simulink model "control_pos_3dof_sinMI"  (R2023b)
settings: Solver=ode5  StartTime=0.0  StopTime=tsim  FixedStep=tstep  RelTol=1e-3
undefined symbols (not defined in the file): a0, a1, robot_params, t_qeq_init, t_tr_init, tau_L
(part 1 of 2)
settings Model: Creator=HP  LastModifiedBy=HP

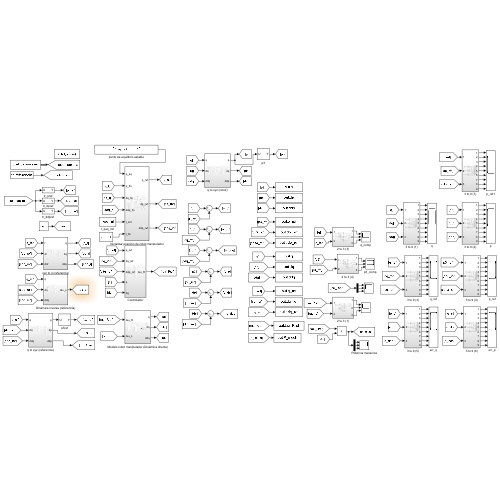
[thumbnail: Simulink's stored preview of the top-level diagram]
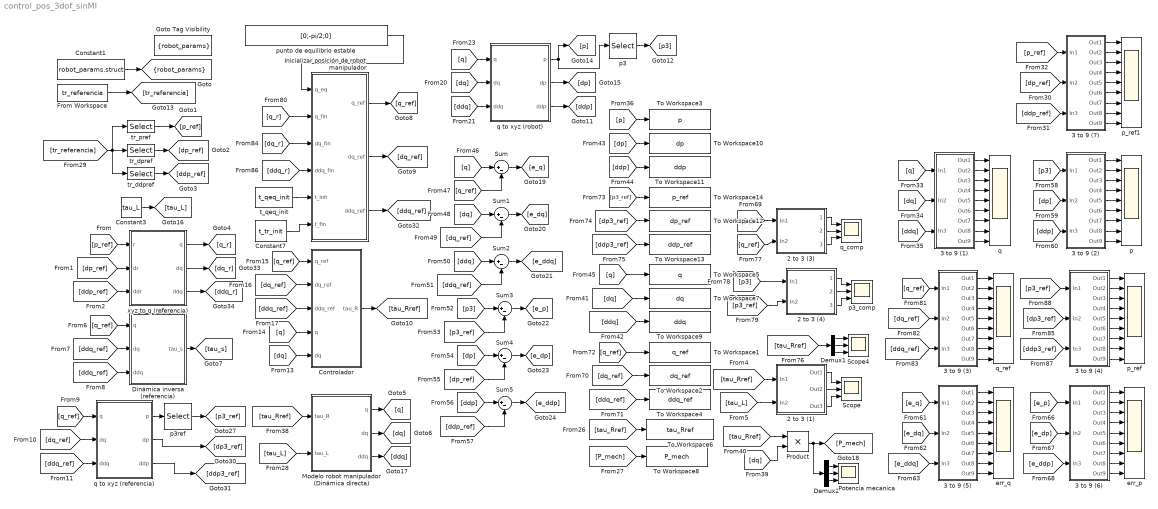
== system control_pos_3dof_sinMI ==
  2 to 3 (1) : Subsystem
  2 to 3 (3) : Subsystem
  2 to 3 (4) : Subsystem
  3 to 9 (1) : Subsystem
  3 to 9 (2) : Subsystem
  3 to 9 (3) : Subsystem
  3 to 9 (4) : Subsystem
  3 to 9 (5) : Subsystem
  3 to 9 (6) : Subsystem
  3 to 9 (7) : Subsystem
  Constant1 : Constant  Value=robot_params.struct  OutDataTypeStr=Bus: robot_params_bus
  Constant3 : Constant  Value=tau_L
  Constant7 : Constant  Value=t_tr_init
  Controlador : Subsystem
  Demux1 : Demux  Outputs=3
  Demux2 : Demux  Outputs=3
  Dinámica inversa (referencia) : Subsystem
  From Workspace : FromWorkspace  VariableName=tr_referencia
  Goto Tag Visibility : GotoTagVisibility  GotoTag=robot_params
  Inicializar posición de robot manipulador : Subsystem
  Modelo robot manipulador (Dinámica directa) : Subsystem
  Potencia mecanica : Scope  NumInputPorts=3
  Product : Product
  Scope : Scope  NumInputPorts=3
  Scope4 : Scope  NumInputPorts=3
  Sum{,1..5} (6 alike) : Sum  Inputs=|+-
  To Workspace1 : ToWorkspace  VariableName=q_ref  SaveFormat=Timeseries  SampleTime=-1
  To Workspace10 : ToWorkspace  VariableName=dp  SaveFormat=Timeseries  SampleTime=-1
  To Workspace11 : ToWorkspace  VariableName=ddp  SaveFormat=Timeseries  SampleTime=-1
  To Workspace12 : ToWorkspace  VariableName=dp_ref  SaveFormat=Timeseries  SampleTime=-1
  To Workspace13 : ToWorkspace  VariableName=ddp_ref  SaveFormat=Timeseries  SampleTime=-1
  To Workspace14 : ToWorkspace  VariableName=p_ref  SaveFormat=Timeseries  SampleTime=-1
  To Workspace2 : ToWorkspace  VariableName=dq_ref  SaveFormat=Timeseries  SampleTime=-1
  To Workspace3 : ToWorkspace  VariableName=p  SaveFormat=Timeseries  SampleTime=-1
  To Workspace4 : ToWorkspace  VariableName=ddq_ref  SaveFormat=Timeseries  SampleTime=-1
  To Workspace5 : ToWorkspace  VariableName=q  SaveFormat=Timeseries  SampleTime=-1
  To Workspace6 : ToWorkspace  VariableName=tau_Rref  SaveFormat=Timeseries  SampleTime=-1
  To Workspace7 : ToWorkspace  VariableName=dq  SaveFormat=Timeseries  SampleTime=-1
  To Workspace8 : ToWorkspace  VariableName=P_mech  SaveFormat=Timeseries  SampleTime=-1
  To Workspace9 : ToWorkspace  VariableName=ddq  SaveFormat=Timeseries  SampleTime=-1
  err_p : Scope  NumInputPorts=9
  err_q : Scope  NumInputPorts=9
  p : Scope  NumInputPorts=9
  p3 : Selector  NumberOfDimensions=2  InputPortWidth=3  IndexOptions=Index vector (dialog),Index vector (dialog)  Indices=[1:3],3  OutputSizes=1,1
  p3_comp : Scope  NumInputPorts=3
  p3ref : Selector  NumberOfDimensions=2  InputPortWidth=3  IndexOptions=Index vector (dialog),Index vector (dialog)  Indices=[1:3],3  OutputSizes=1,1
  p_ref : Scope  NumInputPorts=9
  p_ref1 : Scope  NumInputPorts=9
  punto de equilibrio estable : Constant  Value=[0;-pi/2;0]
  q : Scope  NumInputPorts=9
  q to xyz (referencia) : Subsystem
  q to xyz (robot) : Subsystem
  q_comp : Scope  NumInputPorts=3
  q_ref : Scope  NumInputPorts=9
  t_qeq_init : Constant  Value=t_qeq_init
  tr_ddpref : Selector  NumberOfDimensions=2  InputPortWidth=3  IndexOptions=Index vector (dialog),Index vector (dialog)  Indices=[7:9],1  OutputSizes=1,1
  tr_dpref : Selector  NumberOfDimensions=2  InputPortWidth=3  IndexOptions=Index vector (dialog),Index vector (dialog)  Indices=[4:6],1  OutputSizes=1,1
  tr_pref : Selector  NumberOfDimensions=2  InputPortWidth=3  IndexOptions=Index vector (dialog),Index vector (dialog)  Indices=[1:3],1  OutputSizes=1,1
  xyz to q (referencia) : Subsystem
  tag scope: robot_params=scoped
  wires:
  From Workspace/1 -> [tr_referencia]
  Constant1/1 -> [robot_params]
  Constant3/1 -> [tau_L]
  [q_ref] -> Dinámica inversa (referencia)/1(q)
  [ddq_ref] -> Dinámica inversa (referencia)/2(dq)
  [ddq_ref] -> Dinámica inversa (referencia)/3(ddq)
  Dinámica inversa (referencia)/1(tau_s) -> [tau_s]
  [q_ref] -> Controlador/1(q_ref)
  [dq_ref] -> Controlador/2(dq_ref)
  [ddq_ref] -> Controlador/3(ddq_ref)
  [q] -> Controlador/4(q)
  [dq] -> Controlador/5(dq)
  Controlador/1(tau_R) -> [tau_Rref]
  [tr_referencia] -> tr_ddpref/1, tr_pref/1, tr_dpref/1
  tr_pref/1 -> [p_ref]
  tr_dpref/1 -> [dp_ref]
  tr_ddpref/1 -> [ddp_ref]
  3 to 9 (5)/3(Out3) -> err_q/3
  3 to 9 (2)/5(Out5) -> p/5
  3 to 9 (3)/9(Out9) -> q_ref/9
  3 to 9 (6)/5(Out5) -> err_p/5
  3 to 9 (5)/4(Out4) -> err_q/4
  3 to 9 (7)/8(Out8) -> p_ref1/8
  3 to 9 (4)/3(Out3) -> p_ref/3
  3 to 9 (1)/1(Out1) -> q/1
  [dp3_ref] -> 3 to 9 (4)/2(In2)
  3 to 9 (3)/2(Out2) -> q_ref/2
  [dq] -> To Workspace7/1
  2 to 3 (4)/2(2) -> p3_comp/2
  [ddq_ref] -> 3 to 9 (3)/3(In3)
  [dp] -> Sum4/1
  3 to 9 (1)/9(Out9) -> q/9
  [ddp] -> 3 to 9 (2)/3(In3)
  3 to 9 (2)/8(Out8) -> p/8
  3 to 9 (2)/1(Out1) -> p/1
  [dp] -> 3 to 9 (2)/2(In2)
  [q_ref] -> 2 to 3 (3)/2(In2)
  2 to 3 (3)/2(2) -> q_comp/2
  3 to 9 (4)/5(Out5) -> p_ref/5
  [q] -> 2 to 3 (3)/1(In1)
  [ddp_ref] -> 3 to 9 (7)/3(In3)
  [ddq] -> 3 to 9 (1)/3(In3)
  3 to 9 (2)/3(Out3) -> p/3
  3 to 9 (1)/2(Out2) -> q/2
  3 to 9 (2)/4(Out4) -> p/4
  3 to 9 (4)/6(Out6) -> p_ref/6
  3 to 9 (6)/1(Out1) -> err_p/1
  [p3_ref] -> 3 to 9 (4)/1(In1)
  3 to 9 (1)/3(Out3) -> q/3
  [ddp3_ref] -> 3 to 9 (4)/3(In3)
  3 to 9 (1)/8(Out8) -> q/8
  3 to 9 (7)/9(Out9) -> p_ref1/9
  3 to 9 (7)/1(Out1) -> p_ref1/1
  3 to 9 (4)/4(Out4) -> p_ref/4
  3 to 9 (5)/1(Out1) -> err_q/1
  3 to 9 (2)/2(Out2) -> p/2
  3 to 9 (6)/4(Out4) -> err_p/4
  [ddp] -> Sum5/1
  3 to 9 (7)/3(Out3) -> p_ref1/3
  [q] -> q to xyz (robot)/1(q)
  3 to 9 (3)/4(Out4) -> q_ref/4
  3 to 9 (7)/5(Out5) -> p_ref1/5
  2 to 3 (3)/1(1) -> q_comp/1
  3 to 9 (4)/7(Out7) -> p_ref/7
  [e_ddq] -> 3 to 9 (5)/3(In3)
  3 to 9 (1)/4(Out4) -> q/4
  3 to 9 (3)/3(Out3) -> q_ref/3
  [q_ref] -> To Workspace1/1
  3 to 9 (3)/5(Out5) -> q_ref/5
  [P_mech] -> To Workspace8/1
  3 to 9 (5)/6(Out6) -> err_q/6
  2 to 3 (4)/1(1) -> p3_comp/1
  3 to 9 (6)/7(Out7) -> err_p/7
  [e_q] -> 3 to 9 (5)/1(In1)
  3 to 9 (4)/1(Out1) -> p_ref/1
  3 to 9 (5)/8(Out8) -> err_q/8
  [tau_Rref] -> Demux1/1
  3 to 9 (2)/7(Out7) -> p/7
  Sum5/1 -> [e_ddp]
  Demux2/3 -> Potencia mecanica/3
  3 to 9 (4)/8(Out8) -> p_ref/8
  3 to 9 (6)/2(Out2) -> err_p/2
  [tau_Rref] -> To Workspace6/1
  [e_dp] -> 3 to 9 (6)/2(In2)
  [p3] -> 2 to 3 (4)/1(In1)
  3 to 9 (5)/7(Out7) -> err_q/7
  3 to 9 (3)/1(Out1) -> q_ref/1
  [ddq] -> Sum2/1
  3 to 9 (2)/9(Out9) -> p/9
  3 to 9 (3)/6(Out6) -> q_ref/6
  3 to 9 (4)/9(Out9) -> p_ref/9
  3 to 9 (3)/8(Out8) -> q_ref/8
  3 to 9 (1)/7(Out7) -> q/7
  [ddq_ref] -> Sum2/2
  [dp3_ref] -> To Workspace12/1
  2 to 3 (1)/3(Out3) -> Scope/3
  2 to 3 (4)/3(3) -> p3_comp/3
  3 to 9 (4)/2(Out2) -> p_ref/2
  [dq_ref] -> 3 to 9 (3)/2(In2)
  3 to 9 (6)/3(Out3) -> err_p/3
  [dq] -> Product/2
  3 to 9 (5)/5(Out5) -> err_q/5
  [e_p] -> 3 to 9 (6)/1(In1)
  [dq] -> 3 to 9 (1)/2(In2)
  [dq] -> Sum1/1
  [p_ref] -> 3 to 9 (7)/1(In1)
  Sum/1 -> [e_q]
  3 to 9 (5)/9(Out9) -> err_q/9
  3 to 9 (7)/4(Out4) -> p_ref1/4
  3 to 9 (7)/6(Out6) -> p_ref1/6
  [dp_ref] -> 3 to 9 (7)/2(In2)
  Demux1/1 -> Scope4/1
  2 to 3 (3)/3(3) -> q_comp/3
  [q_ref] -> 3 to 9 (3)/1(In1)
  Sum2/1 -> [e_ddq]
  Demux1/2 -> Scope4/2
  [tau_L] -> 2 to 3 (1)/2(In2)
  Demux2/2 -> Potencia mecanica/2
  [p3] -> 3 to 9 (2)/1(In1)
  q to xyz (robot)/1(p) -> p3/1, [p]
  3 to 9 (6)/8(Out8) -> err_p/8
  [q_ref] -> Sum/2
  3 to 9 (6)/6(Out6) -> err_p/6
  3 to 9 (1)/6(Out6) -> q/6
  [dp] -> To Workspace10/1
  Demux1/3 -> Scope4/3
  3 to 9 (7)/7(Out7) -> p_ref1/7
  [p] -> To Workspace3/1
  [ddq_ref] -> To Workspace4/1
  Sum3/1 -> [e_p]
  Sum4/1 -> [e_dp]
  [p3] -> Sum3/1
  [dq_ref] -> Sum1/2
  3 to 9 (2)/6(Out6) -> p/6
  Sum1/1 -> [e_dq]
  [tau_Rref] -> 2 to 3 (1)/1(In1)
  Demux2/1 -> Potencia mecanica/1
  [e_dq] -> 3 to 9 (5)/2(In2)
  [q] -> Sum/1
  [dp_ref] -> Sum4/2
  3 to 9 (5)/2(Out2) -> err_q/2
  [ddq] -> q to xyz (robot)/3(ddq)
  [e_ddp] -> 3 to 9 (6)/3(In3)
  [ddp_ref] -> Sum5/2
  [p3_ref] -> Sum3/2
  3 to 9 (3)/7(Out7) -> q_ref/7
  [p3_ref] -> 2 to 3 (4)/2(In2)
  p3/1 -> [p3]
  2 to 3 (1)/1(Out1) -> Scope/1
  [dq] -> q to xyz (robot)/2(dq)
  [ddp3_ref] -> To Workspace13/1
  3 to 9 (1)/5(Out5) -> q/5
  [ddq] -> To Workspace9/1
  [p3_ref] -> To Workspace14/1
  [ddp] -> To Workspace11/1
  3 to 9 (6)/9(Out9) -> err_p/9
  q to xyz (robot)/3(ddp) -> [ddp]
  [q] -> 3 to 9 (1)/1(In1)
  [q] -> To Workspace5/1
  q to xyz (robot)/2(dp) -> [dp]
  [dq_ref] -> To Workspace2/1
  Product/1 -> Demux2/1, [P_mech]
  [tau_Rref] -> Product/1
  3 to 9 (7)/2(Out2) -> p_ref1/2
  2 to 3 (1)/2(Out2) -> Scope/2
  xyz to q (referencia)/1(q) -> [q_r]
  xyz to q (referencia)/2(dq) -> [dq_r]
  [ddp_ref] -> xyz to q (referencia)/3(ddr)
  [p_ref] -> xyz to q (referencia)/1(r)
  [dp_ref] -> xyz to q (referencia)/2(dr)
  xyz to q (referencia)/3(ddq) -> [ddq_r]
  [dq_ref] -> q to xyz (referencia)/2(dq)
  q to xyz (referencia)/2(dp) -> [dp3_ref]
  q to xyz (referencia)/3(ddp) -> [ddp3_ref]
  [ddq_ref] -> q to xyz (referencia)/3(ddq)
  Modelo robot manipulador (Dinámica directa)/3(ddq) -> [ddq]
  [tau_L] -> Modelo robot manipulador (Dinámica directa)/2(tau_L)
  Modelo robot manipulador (Dinámica directa)/1(q) -> [q]
  Modelo robot manipulador (Dinámica directa)/2(dq) -> [dq]
  [tau_Rref] -> Modelo robot manipulador (Dinámica directa)/1(tau_R)
  [q_ref] -> q to xyz (referencia)/1(q)
  q to xyz (referencia)/1(p) -> p3ref/1
  p3ref/1 -> [p3_ref]
  Constant7/1 -> Inicializar posición de robot manipulador/6(t_fin)
  [dq_r] -> Inicializar posición de robot manipulador/3(dq_fin)
  [q_r] -> Inicializar posición de robot manipulador/2(q_fin)
  [ddq_r] -> Inicializar posición de robot manipulador/4(ddq_fin)
  t_qeq_init/1 -> Inicializar posición de robot manipulador/5(t_init)
  Inicializar posición de robot manipulador/3(ddq_ref) -> [ddq_ref]
  punto de equilibrio estable/1 -> Inicializar posición de robot manipulador/1(q_eq)
  Inicializar posición de robot manipulador/1(q_ref) -> [q_ref]
  Inicializar posición de robot manipulador/2(dq_ref) -> [dq_ref]

== system control_pos_3dof_sinMI/2 to 3 (1) ==
  In1 : Inport
  In2 : Inport  Port=2
  Demux : Demux  Outputs=3
  Demux1 : Demux  Outputs=3
  Mux : Mux  Inputs=2
  Mux1 : Mux  Inputs=2
  Mux2 : Mux  Inputs=2
  Out1 : Outport
  Out2 : Outport  Port=2
  Out3 : Outport  Port=3
  wires:
  Demux/3 -> Mux2/1
  Mux2/1 -> Out3/1
  Mux1/1 -> Out2/1
  Demux/1 -> Mux/1
  Demux1/1 -> Mux/2
  In1/1 -> Demux/1
  Demux/2 -> Mux1/1
  Demux1/2 -> Mux1/2
  Mux/1 -> Out1/1
  Demux1/3 -> Mux2/2
  In2/1 -> Demux1/1

== system control_pos_3dof_sinMI/2 to 3 (3) ==
  In1 : Inport
  In2 : Inport  Port=2
  Demux3 : Demux  Outputs=3
  Demux4 : Demux  Outputs=3
  Mux10 : Mux  Inputs=2
  Mux8 : Mux  Inputs=2
  Mux9 : Mux  Inputs=2
  1 : Outport
  2 : Outport  Port=2
  3 : Outport  Port=3
  wires:
  Demux4/3 -> Mux10/2
  Demux3/1 -> Mux8/1
  Demux3/2 -> Mux9/1
  Mux9/1 -> 2/1
  Demux4/2 -> Mux9/2
  Demux4/1 -> Mux8/2
  Demux3/3 -> Mux10/1
  Mux8/1 -> 1/1
  Mux10/1 -> 3/1
  In1/1 -> Demux3/1
  In2/1 -> Demux4/1

== system control_pos_3dof_sinMI/2 to 3 (4) ==
  In1 : Inport
  In2 : Inport  Port=2
  Demux3 : Demux  Outputs=3
  Demux4 : Demux  Outputs=3
  Mux10 : Mux  Inputs=2
  Mux8 : Mux  Inputs=2
  Mux9 : Mux  Inputs=2
  1 : Outport
  2 : Outport  Port=2
  3 : Outport  Port=3
  wires:
  Demux4/3 -> Mux10/2
  Demux3/1 -> Mux8/1
  Demux3/2 -> Mux9/1
  Mux9/1 -> 2/1
  Demux4/2 -> Mux9/2
  Demux4/1 -> Mux8/2
  Demux3/3 -> Mux10/1
  Mux8/1 -> 1/1
  Mux10/1 -> 3/1
  In1/1 -> Demux3/1
  In2/1 -> Demux4/1

== system control_pos_3dof_sinMI/3 to 9 (1) ==
  In1 : Inport
  In2 : Inport  Port=2
  In3 : Inport  Port=3
  Demux2 : Demux  Outputs=3
  Demux3 : Demux  Outputs=3
  Demux4 : Demux  Outputs=3
  Out1 : Outport
  Out2 : Outport  Port=2
  Out3 : Outport  Port=3
  Out4 : Outport  Port=4
  Out5 : Outport  Port=5
  Out6 : Outport  Port=6
  Out7 : Outport  Port=7
  Out8 : Outport  Port=8
  Out9 : Outport  Port=9
  wires:
  In3/1 -> Demux4/1
  Demux4/1 -> Out3/1
  Demux2/1 -> Out1/1
  Demux3/3 -> Out8/1
  Demux3/2 -> Out5/1
  Demux3/1 -> Out2/1
  In1/1 -> Demux2/1
  Demux2/3 -> Out7/1
  Demux4/3 -> Out9/1
  Demux4/2 -> Out6/1
  Demux2/2 -> Out4/1
  In2/1 -> Demux3/1

== system control_pos_3dof_sinMI/3 to 9 (2) ==
  In1 : Inport
  In2 : Inport  Port=2
  In3 : Inport  Port=3
  Demux2 : Demux  Outputs=3
  Demux3 : Demux  Outputs=3
  Demux4 : Demux  Outputs=3
  Out1 : Outport
  Out2 : Outport  Port=2
  Out3 : Outport  Port=3
  Out4 : Outport  Port=4
  Out5 : Outport  Port=5
  Out6 : Outport  Port=6
  Out7 : Outport  Port=7
  Out8 : Outport  Port=8
  Out9 : Outport  Port=9
  wires:
  In3/1 -> Demux4/1
  Demux4/1 -> Out3/1
  Demux2/1 -> Out1/1
  Demux3/3 -> Out8/1
  Demux3/2 -> Out5/1
  Demux3/1 -> Out2/1
  In1/1 -> Demux2/1
  Demux2/3 -> Out7/1
  Demux4/3 -> Out9/1
  Demux4/2 -> Out6/1
  Demux2/2 -> Out4/1
  In2/1 -> Demux3/1

== system control_pos_3dof_sinMI/3 to 9 (3) ==
  In1 : Inport
  In2 : Inport  Port=2
  In3 : Inport  Port=3
  Demux2 : Demux  Outputs=3
  Demux3 : Demux  Outputs=3
  Demux4 : Demux  Outputs=3
  Out1 : Outport
  Out2 : Outport  Port=2
  Out3 : Outport  Port=3
  Out4 : Outport  Port=4
  Out5 : Outport  Port=5
  Out6 : Outport  Port=6
  Out7 : Outport  Port=7
  Out8 : Outport  Port=8
  Out9 : Outport  Port=9
  wires:
  In3/1 -> Demux4/1
  Demux4/1 -> Out3/1
  Demux2/1 -> Out1/1
  Demux3/3 -> Out8/1
  Demux3/2 -> Out5/1
  Demux3/1 -> Out2/1
  In1/1 -> Demux2/1
  Demux2/3 -> Out7/1
  Demux4/3 -> Out9/1
  Demux4/2 -> Out6/1
  Demux2/2 -> Out4/1
  In2/1 -> Demux3/1

== system control_pos_3dof_sinMI/3 to 9 (4) ==
  In1 : Inport
  In2 : Inport  Port=2
  In3 : Inport  Port=3
  Demux2 : Demux  Outputs=3
  Demux3 : Demux  Outputs=3
  Demux4 : Demux  Outputs=3
  Out1 : Outport
  Out2 : Outport  Port=2
  Out3 : Outport  Port=3
  Out4 : Outport  Port=4
  Out5 : Outport  Port=5
  Out6 : Outport  Port=6
  Out7 : Outport  Port=7
  Out8 : Outport  Port=8
  Out9 : Outport  Port=9
  wires:
  In3/1 -> Demux4/1
  Demux4/1 -> Out3/1
  Demux2/1 -> Out1/1
  Demux3/3 -> Out8/1
  Demux3/2 -> Out5/1
  Demux3/1 -> Out2/1
  In1/1 -> Demux2/1
  Demux2/3 -> Out7/1
  Demux4/3 -> Out9/1
  Demux4/2 -> Out6/1
  Demux2/2 -> Out4/1
  In2/1 -> Demux3/1

== system control_pos_3dof_sinMI/3 to 9 (5) ==
  In1 : Inport
  In2 : Inport  Port=2
  In3 : Inport  Port=3
  Demux2 : Demux  Outputs=3
  Demux3 : Demux  Outputs=3
  Demux4 : Demux  Outputs=3
  Out1 : Outport
  Out2 : Outport  Port=2
  Out3 : Outport  Port=3
  Out4 : Outport  Port=4
  Out5 : Outport  Port=5
  Out6 : Outport  Port=6
  Out7 : Outport  Port=7
  Out8 : Outport  Port=8
  Out9 : Outport  Port=9
  wires:
  In3/1 -> Demux4/1
  Demux4/1 -> Out3/1
  Demux2/1 -> Out1/1
  Demux3/3 -> Out8/1
  Demux3/2 -> Out5/1
  Demux3/1 -> Out2/1
  In1/1 -> Demux2/1
  Demux2/3 -> Out7/1
  Demux4/3 -> Out9/1
  Demux4/2 -> Out6/1
  Demux2/2 -> Out4/1
  In2/1 -> Demux3/1

== system control_pos_3dof_sinMI/3 to 9 (6) ==
  In1 : Inport
  In2 : Inport  Port=2
  In3 : Inport  Port=3
  Demux2 : Demux  Outputs=3
  Demux3 : Demux  Outputs=3
  Demux4 : Demux  Outputs=3
  Out1 : Outport
  Out2 : Outport  Port=2
  Out3 : Outport  Port=3
  Out4 : Outport  Port=4
  Out5 : Outport  Port=5
  Out6 : Outport  Port=6
  Out7 : Outport  Port=7
  Out8 : Outport  Port=8
  Out9 : Outport  Port=9
  wires:
  In3/1 -> Demux4/1
  Demux4/1 -> Out3/1
  Demux2/1 -> Out1/1
  Demux3/3 -> Out8/1
  Demux3/2 -> Out5/1
  Demux3/1 -> Out2/1
  In1/1 -> Demux2/1
  Demux2/3 -> Out7/1
  Demux4/3 -> Out9/1
  Demux4/2 -> Out6/1
  Demux2/2 -> Out4/1
  In2/1 -> Demux3/1

== system control_pos_3dof_sinMI/3 to 9 (7) ==
  In1 : Inport
  In2 : Inport  Port=2
  In3 : Inport  Port=3
  Demux2 : Demux  Outputs=3
  Demux3 : Demux  Outputs=3
  Demux4 : Demux  Outputs=3
  Out1 : Outport
  Out2 : Outport  Port=2
  Out3 : Outport  Port=3
  Out4 : Outport  Port=4
  Out5 : Outport  Port=5
  Out6 : Outport  Port=6
  Out7 : Outport  Port=7
  Out8 : Outport  Port=8
  Out9 : Outport  Port=9
  wires:
  In3/1 -> Demux4/1
  Demux4/1 -> Out3/1
  Demux2/1 -> Out1/1
  Demux3/3 -> Out8/1
  Demux3/2 -> Out5/1
  Demux3/1 -> Out2/1
  In1/1 -> Demux2/1
  Demux2/3 -> Out7/1
  Demux4/3 -> Out9/1
  Demux4/2 -> Out6/1
  Demux2/2 -> Out4/1
  In2/1 -> Demux3/1

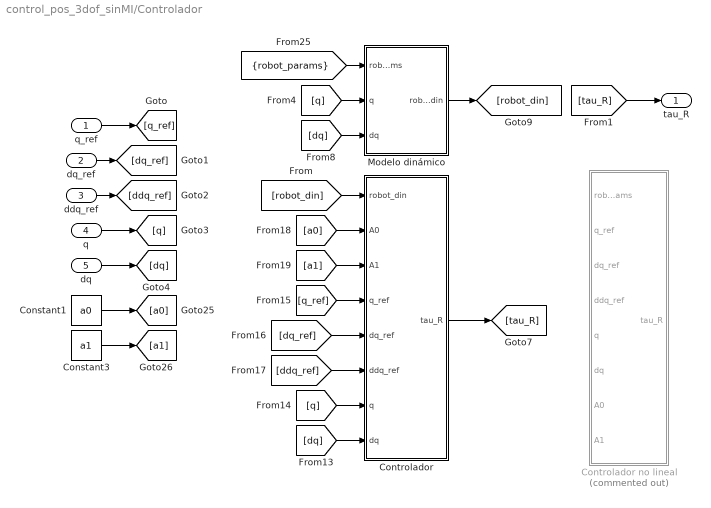
== system control_pos_3dof_sinMI/Controlador ==
  q_ref : Inport
  dq_ref : Inport  Port=2
  ddq_ref : Inport  Port=3
  q : Inport  Port=4
  dq : Inport  Port=5
  Constant1 : Constant  Value=a0
  Constant3 : Constant  Value=a1
  Controlador : MATLAB Function  TreatAsAtomicUnit=on
  Controlador no lineal : MATLAB Function  Commented=on  TreatAsAtomicUnit=on
  Modelo dinámico : MATLAB Function  TreatAsAtomicUnit=on
  tau_R : Outport
  wires:
  [dq] -> Modelo dinámico/3(dq)
  [q] -> Modelo dinámico/2(q)
  [robot_params] -> Modelo dinámico/1(robot_params)
  Modelo dinámico/1(robot_din) -> [robot_din]
  dq/1 -> [dq]
  q/1 -> [q]
  ddq_ref/1 -> [ddq_ref]
  dq_ref/1 -> [dq_ref]
  q_ref/1 -> [q_ref]
  [robot_din] -> Controlador/1(robot_din)
  [a0] -> Controlador/2(A0)
  [a1] -> Controlador/3(A1)
  [q_ref] -> Controlador/4(q_ref)
  [dq_ref] -> Controlador/5(dq_ref)
  [ddq_ref] -> Controlador/6(ddq_ref)
  [q] -> Controlador/7(q)
  [dq] -> Controlador/8(dq)
  Controlador/1(tau_R) -> [tau_R]
  [tau_R] -> tau_R/1
  Constant1/1 -> [a0]
  Constant3/1 -> [a1]

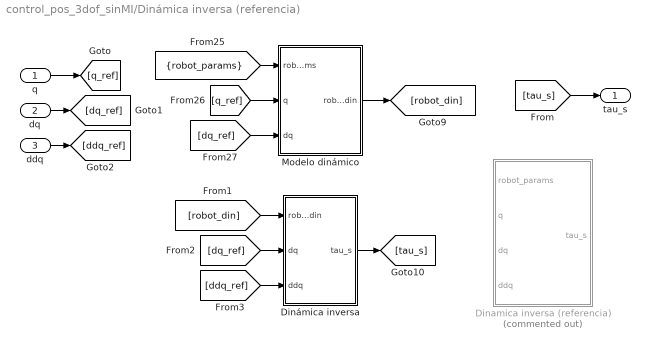
== system control_pos_3dof_sinMI/Dinámica inversa (referencia) ==
  q : Inport
  dq : Inport  Port=2
  ddq : Inport  Port=3
  Dinamica inversa (referencia) : MATLAB Function  Commented=on  TreatAsAtomicUnit=on
  Dinámica inversa : MATLAB Function  TreatAsAtomicUnit=on
  Modelo dinámico : MATLAB Function  TreatAsAtomicUnit=on
  tau_s : Outport
  wires:
  [dq_ref] -> Modelo dinámico/3(dq)
  [robot_params] -> Modelo dinámico/1(robot_params)
  Modelo dinámico/1(robot_din) -> [robot_din]
  [q_ref] -> Modelo dinámico/2(q)
  q/1 -> [q_ref]
  dq/1 -> [dq_ref]
  Dinámica inversa/1(tau_s) -> [tau_s]
  [robot_din] -> Dinámica inversa/1(robot_din)
  [ddq_ref] -> Dinámica inversa/3(ddq)
  [dq_ref] -> Dinámica inversa/2(dq)
  ddq/1 -> [ddq_ref]
  [tau_s] -> tau_s/1

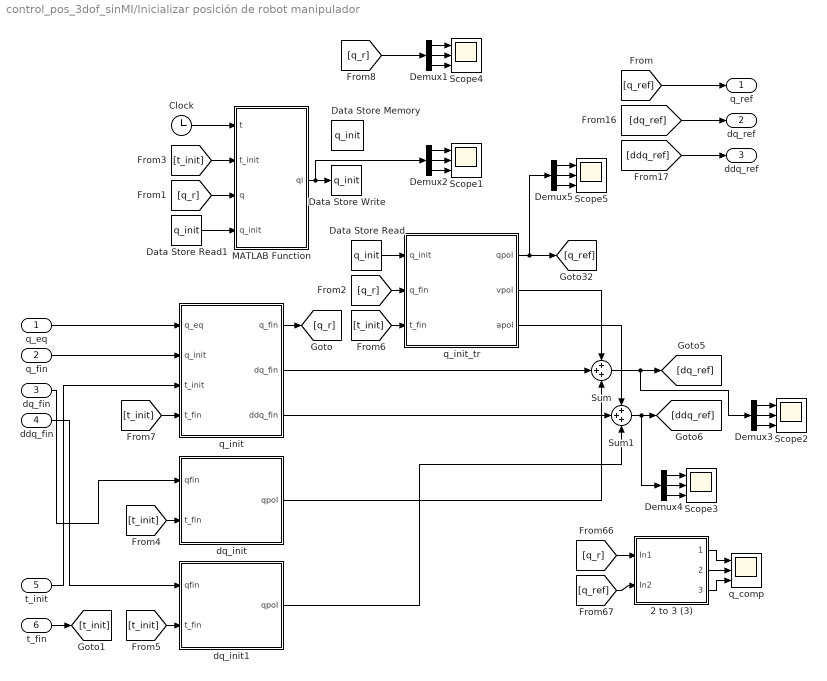
== system control_pos_3dof_sinMI/Inicializar posición de robot manipulador ==
  q_eq : Inport
  q_fin : Inport  Port=2
  dq_fin : Inport  Port=3
  ddq_fin : Inport  Port=4
  t_init : Inport  Port=5
  t_fin : Inport  Port=6
  2 to 3 (3) : Subsystem
  Clock : Clock
  Data Store Memory : DataStoreMemory  DataStoreName=q_init  WriteAfterWriteMsg=warning  InitialValue=[0;-pi/2;0]  ShowAdditionalParam=off
  Data Store Read : DataStoreRead  DataStoreName=q_init  IndexOptions=Index vector (dialog)  Indices=1  OutputSizes=1
  Data Store Read1 : DataStoreRead  DataStoreName=q_init  IndexOptions=Index vector (dialog)  Indices=1  OutputSizes=1
  Data Store Write : DataStoreWrite  DataStoreName=q_init  IndexOptions=Index vector (dialog)  Indices=1  OutputSizes=1
  Demux{1..5} (5 alike) : Demux  Outputs=3
  MATLAB Function : MATLAB Function  TreatAsAtomicUnit=on
  Scope{1..5} (5 alike) : Scope  NumInputPorts=3
  Sum : Sum  Inputs=+++
  Sum1 : Sum  Inputs=+++
  dq_init : Subsystem
  dq_init1 : Subsystem
  q_comp : Scope  NumInputPorts=3
  q_init : Subsystem
  q_init_tr : Subsystem
  q_ref : Outport
  dq_ref : Outport  Port=2
  ddq_ref : Outport  Port=3
  wires:
  [ddq_ref] -> ddq_ref/1
  q_fin/1 -> q_init/2(q_init)
  [t_init] -> dq_init/2(t_fin)
  dq_fin/1 -> dq_init/1(qfin)
  [t_init] -> dq_init1/2(t_fin)
  [dq_ref] -> dq_ref/1
  q_eq/1 -> q_init/1(q_eq)
  ddq_fin/1 -> dq_init1/1(qfin)
  [q_ref] -> q_ref/1
  Sum/1 -> Demux3/1, [dq_ref]
  Sum1/1 -> Demux4/1, [ddq_ref]
  q_init_tr/1(qpol) -> Demux5/1, [q_ref]
  [t_init] -> q_init_tr/3(t_fin)
  [t_init] -> MATLAB Function/2(t_init)
  Clock/1 -> MATLAB Function/1(t)
  MATLAB Function/1(qi) -> Demux2/1, Data Store Write/1
  Data Store Read/1 -> q_init_tr/1(q_init)
  Data Store Read1/1 -> MATLAB Function/4(q_init)
  q_init/1(q_fin) -> [q_r]
  [q_r] -> MATLAB Function/3(q)
  [q_r] -> q_init_tr/2(q_fin)
  t_init/1 -> q_init/3(t_init)
  [q_r] -> Demux1/1
  t_fin/1 -> [t_init]
  [t_init] -> q_init/4(t_fin)
  q_init/2(dq_fin) -> Sum/2
  q_init_tr/2(vpol) -> Sum/1
  dq_init/1(qpol) -> Sum/3
  q_init_tr/3(apol) -> Sum1/1
  q_init/3(ddq_fin) -> Sum1/2
  dq_init1/1(qpol) -> Sum1/3
  [q_ref] -> 2 to 3 (3)/2(In2)
  2 to 3 (3)/2(2) -> q_comp/2
  [q_r] -> 2 to 3 (3)/1(In1)
  2 to 3 (3)/3(3) -> q_comp/3
  2 to 3 (3)/1(1) -> q_comp/1
  Demux1/3 -> Scope4/3
  Demux1/1 -> Scope4/1
  Demux1/2 -> Scope4/2
  Demux2/3 -> Scope1/3
  Demux2/1 -> Scope1/1
  Demux2/2 -> Scope1/2
  Demux3/3 -> Scope2/3
  Demux3/1 -> Scope2/1
  Demux3/2 -> Scope2/2
  Demux4/3 -> Scope3/3
  Demux4/1 -> Scope3/1
  Demux4/2 -> Scope3/2
  Demux5/3 -> Scope5/3
  Demux5/1 -> Scope5/1
  Demux5/2 -> Scope5/2

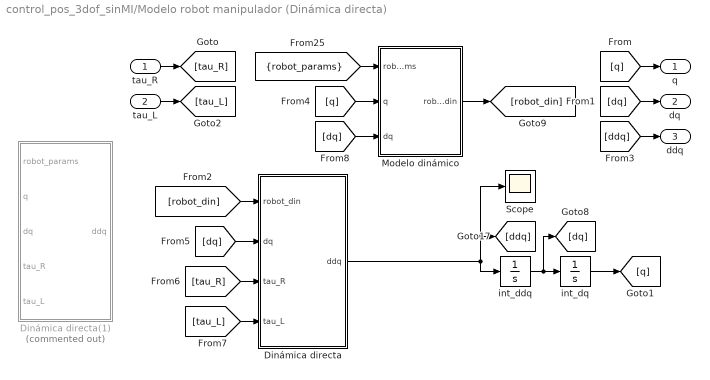
== system control_pos_3dof_sinMI/Modelo robot manipulador (Dinámica directa) ==
  tau_R : Inport
  tau_L : Inport  Port=2
  Dinámica directa : MATLAB Function  TreatAsAtomicUnit=on
  Dinámica directa(1) : MATLAB Function  Commented=on  TreatAsAtomicUnit=on
  Modelo dinámico : MATLAB Function  TreatAsAtomicUnit=on
  Scope : Scope
  int_ddq : Integrator  InitialCondition=[0;0;0]
  int_dq : Integrator  InitialCondition=[0;-1.5708;0]
  q : Outport
  dq : Outport  Port=2
  ddq : Outport  Port=3
  wires:
  [robot_params] -> Modelo dinámico/1(robot_params)
  [dq] -> Modelo dinámico/3(dq)
  Modelo dinámico/1(robot_din) -> [robot_din]
  [q] -> Modelo dinámico/2(q)
  [tau_L] -> Dinámica directa/4(tau_L)
  int_ddq/1 -> [dq], int_dq/1
  [robot_din] -> Dinámica directa/1(robot_din)
  [dq] -> Dinámica directa/2(dq)
  int_dq/1 -> [q]
  [tau_R] -> Dinámica directa/3(tau_R)
  [q] -> q/1
  [dq] -> dq/1
  [ddq] -> ddq/1
  tau_R/1 -> [tau_R]
  tau_L/1 -> [tau_L]
  Dinámica directa/1(ddq) -> Scope/1, [ddq], int_ddq/1

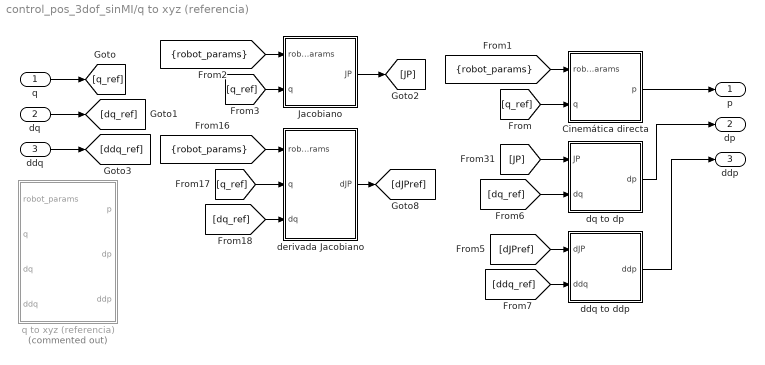
== system control_pos_3dof_sinMI/q to xyz (referencia) ==
  q : Inport
  dq : Inport  Port=2
  ddq : Inport  Port=3
  Cinemática directa : MATLAB Function  TreatAsAtomicUnit=on
  Jacobiano : MATLAB Function  TreatAsAtomicUnit=on
  ddq to ddp : MATLAB Function  TreatAsAtomicUnit=on
  derivada Jacobiano : MATLAB Function  TreatAsAtomicUnit=on
  dq to dp : MATLAB Function  TreatAsAtomicUnit=on
  q to xyz (referencia) : MATLAB Function  Commented=on  TreatAsAtomicUnit=on
  p : Outport
  dp : Outport  Port=2
  ddp : Outport  Port=3
  wires:
  q/1 -> [q_ref]
  ddq/1 -> [ddq_ref]
  dq/1 -> [dq_ref]
  [dq_ref] -> derivada Jacobiano/3(dq)
  derivada Jacobiano/1(dJP) -> [dJPref]
  [robot_params] -> derivada Jacobiano/1(robot_params)
  [q_ref] -> derivada Jacobiano/2(q)
  [q_ref] -> Cinemática directa/2(q)
  [robot_params] -> Cinemática directa/1(robot_params)
  [robot_params] -> Jacobiano/1(robot_params)
  [q_ref] -> Jacobiano/2(q)
  Jacobiano/1(JP) -> [JP]
  dq to dp/1(dp) -> dp/1
  [dq_ref] -> dq to dp/2(dq)
  [dJPref] -> ddq to ddp/1(dJP)
  [JP] -> dq to dp/1(JP)
  ddq to ddp/1(ddp) -> ddp/1
  [ddq_ref] -> ddq to ddp/2(ddq)
  Cinemática directa/1(p) -> p/1

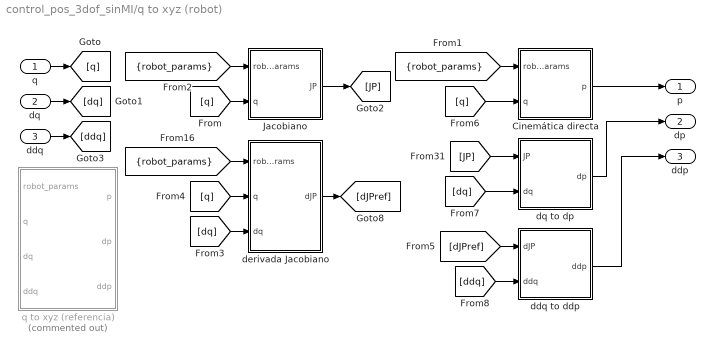
== system control_pos_3dof_sinMI/q to xyz (robot) ==
  q : Inport
  dq : Inport  Port=2
  ddq : Inport  Port=3
  Cinemática directa : MATLAB Function  TreatAsAtomicUnit=on
  Jacobiano : MATLAB Function  TreatAsAtomicUnit=on
  ddq to ddp : MATLAB Function  TreatAsAtomicUnit=on
  derivada Jacobiano : MATLAB Function  TreatAsAtomicUnit=on
  dq to dp : MATLAB Function  TreatAsAtomicUnit=on
  q to xyz (referencia) : MATLAB Function  Commented=on  TreatAsAtomicUnit=on
  p : Outport
  dp : Outport  Port=2
  ddp : Outport  Port=3
  wires:
  q/1 -> [q]
  ddq/1 -> [ddq]
  dq/1 -> [dq]
  [dq] -> derivada Jacobiano/3(dq)
  derivada Jacobiano/1(dJP) -> [dJPref]
  [robot_params] -> derivada Jacobiano/1(robot_params)
  [q] -> derivada Jacobiano/2(q)
  [q] -> Cinemática directa/2(q)
  [robot_params] -> Cinemática directa/1(robot_params)
  [robot_params] -> Jacobiano/1(robot_params)
  [q] -> Jacobiano/2(q)
  Jacobiano/1(JP) -> [JP]
  dq to dp/1(dp) -> dp/1
  [dq] -> dq to dp/2(dq)
  [dJPref] -> ddq to ddp/1(dJP)
  [JP] -> dq to dp/1(JP)
  ddq to ddp/1(ddp) -> ddp/1
  [ddq] -> ddq to ddp/2(ddq)
  Cinemática directa/1(p) -> p/1

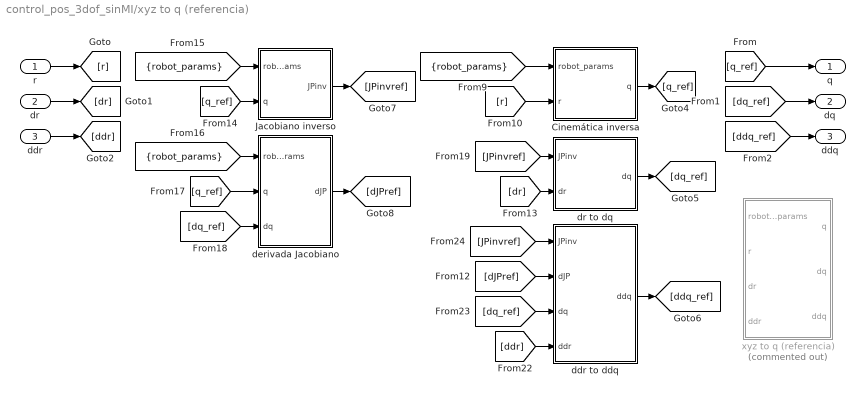
== system control_pos_3dof_sinMI/xyz to q (referencia) ==
  r : Inport
  dr : Inport  Port=2
  ddr : Inport  Port=3
  Cinemática inversa : MATLAB Function  TreatAsAtomicUnit=on
  Jacobiano inverso : MATLAB Function  TreatAsAtomicUnit=on
  ddr to ddq : MATLAB Function  TreatAsAtomicUnit=on
  derivada Jacobiano : MATLAB Function  TreatAsAtomicUnit=on
  dr to dq : MATLAB Function  TreatAsAtomicUnit=on
  xyz to q (referencia) : MATLAB Function  Commented=on  TreatAsAtomicUnit=on
  q : Outport
  dq : Outport  Port=2
  ddq : Outport  Port=3
  wires:
  r/1 -> [r]
  dr/1 -> [dr]
  ddr/1 -> [ddr]
  [robot_params] -> Cinemática inversa/1(robot_params)
  ddr to ddq/1(ddq) -> [ddq_ref]
  [robot_params] -> derivada Jacobiano/1(robot_params)
  [robot_params] -> Jacobiano inverso/1(robot_params)
  dr to dq/1(dq) -> [dq_ref]
  derivada Jacobiano/1(dJP) -> [dJPref]
  [r] -> Cinemática inversa/2(r)
  [dr] -> dr to dq/2(dr)
  [JPinvref] -> dr to dq/1(JPinv)
  [q_ref] -> derivada Jacobiano/2(q)
  [dq_ref] -> derivada Jacobiano/3(dq)
  Jacobiano inverso/1(JPinv) -> [JPinvref]
  [ddr] -> ddr to ddq/4(ddr)
  [JPinvref] -> ddr to ddq/1(JPinv)
  [dq_ref] -> ddr to ddq/3(dq)
  [dJPref] -> ddr to ddq/2(dJP)
  [q_ref] -> Jacobiano inverso/2(q)
  Cinemática inversa/1(q) -> [q_ref]
  [q_ref] -> q/1
  [dq_ref] -> dq/1
  [ddq_ref] -> ddq/1

== system control_pos_3dof_sinMI/Inicializar posición de robot manipulador/2 to 3 (3) ==
  In1 : Inport
  In2 : Inport  Port=2
  Demux3 : Demux  Outputs=3
  Demux4 : Demux  Outputs=3
  Mux10 : Mux  Inputs=2
  Mux8 : Mux  Inputs=2
  Mux9 : Mux  Inputs=2
  1 : Outport
  2 : Outport  Port=2
  3 : Outport  Port=3
  wires:
  Demux4/3 -> Mux10/2
  Demux3/1 -> Mux8/1
  Demux3/2 -> Mux9/1
  Mux9/1 -> 2/1
  Demux4/2 -> Mux9/2
  Demux4/1 -> Mux8/2
  Demux3/3 -> Mux10/1
  Mux8/1 -> 1/1
  Mux10/1 -> 3/1
  In1/1 -> Demux3/1
  In2/1 -> Demux4/1

== system control_pos_3dof_sinMI/Inicializar posición de robot manipulador/dq_init ==
  qfin : Inport
  t_fin : Inport  Port=2
  Demux : Demux  Outputs=3
  Mux : Mux  Inputs=3
  q1 : Subsystem
  q2 : Subsystem
  q3 : Subsystem
  qpol : Outport
  wires:
  qfin/1 -> Demux/1
  t_fin/1 -> [t_fin]
  [t_fin] -> q1/2(t_fin)
  [t_fin] -> q2/2(t_fin)
  [t_fin] -> q3/2(t_fin)
  Mux/1 -> qpol/1
  Demux/1 -> q1/1(q_fin)
  Demux/2 -> q2/1(q_fin)
  Demux/3 -> q3/1(q_fin)
  q1/1(qpol) -> Mux/1
  q2/1(qpol) -> Mux/2
  q3/1(qpol) -> Mux/3

== system control_pos_3dof_sinMI/Inicializar posición de robot manipulador/dq_init1 ==
  qfin : Inport
  t_fin : Inport  Port=2
  Demux : Demux  Outputs=3
  Mux : Mux  Inputs=3
  q1 : Subsystem
  q2 : Subsystem
  q3 : Subsystem
  qpol : Outport
  wires:
  qfin/1 -> Demux/1
  t_fin/1 -> [t_fin]
  [t_fin] -> q1/2(t_fin)
  [t_fin] -> q2/2(t_fin)
  [t_fin] -> q3/2(t_fin)
  Mux/1 -> qpol/1
  Demux/1 -> q1/1(q_fin)
  Demux/2 -> q2/1(q_fin)
  Demux/3 -> q3/1(q_fin)
  q1/1(qpol) -> Mux/1
  q2/1(qpol) -> Mux/2
  q3/1(qpol) -> Mux/3

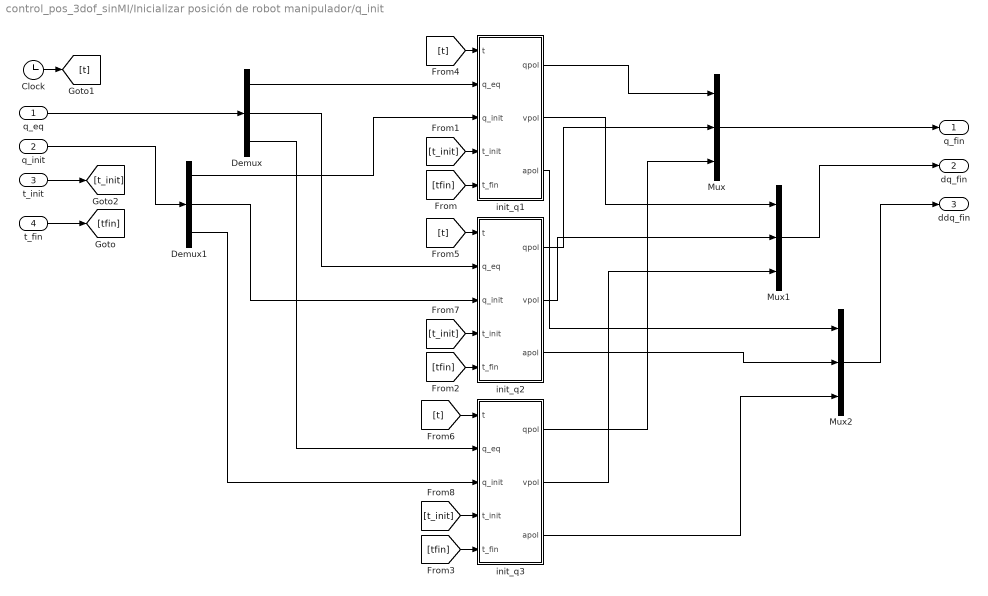
== system control_pos_3dof_sinMI/Inicializar posición de robot manipulador/q_init ==
  q_eq : Inport
  q_init : Inport  Port=2
  t_init : Inport  Port=3
  t_fin : Inport  Port=4
  Clock : Clock
  Demux : Demux  Outputs=3
  Demux1 : Demux  Outputs=3
  Mux : Mux  Inputs=3
  Mux1 : Mux  Inputs=3
  Mux2 : Mux  Inputs=3
  init_q1 : Subsystem
  init_q2 : Subsystem
  init_q3 : Subsystem
  q_fin : Outport
  dq_fin : Outport  Port=2
  ddq_fin : Outport  Port=3
  wires:
  t_fin/1 -> [tfin]
  [tfin] -> init_q1/5(t_fin)
  [tfin] -> init_q2/5(t_fin)
  [tfin] -> init_q3/5(t_fin)
  q_eq/1 -> Demux/1
  q_init/1 -> Demux1/1
  Demux/1 -> init_q1/2(q_eq)
  Demux/2 -> init_q2/2(q_eq)
  [t] -> init_q1/1(t)
  [t] -> init_q2/1(t)
  [t] -> init_q3/1(t)
  Demux/3 -> init_q3/2(q_eq)
  t_init/1 -> [t_init]
  [t_init] -> init_q1/4(t_init)
  [t_init] -> init_q2/4(t_init)
  [t_init] -> init_q3/4(t_init)
  Clock/1 -> [t]
  Demux1/1 -> init_q1/3(q_init)
  Demux1/2 -> init_q2/3(q_init)
  Demux1/3 -> init_q3/3(q_init)
  init_q1/1(qpol) -> Mux/1
  init_q2/1(qpol) -> Mux/2
  init_q3/1(qpol) -> Mux/3
  init_q1/2(vpol) -> Mux1/1
  init_q2/2(vpol) -> Mux1/2
  init_q3/2(vpol) -> Mux1/3
  init_q3/3(apol) -> Mux2/3
  init_q2/3(apol) -> Mux2/2
  init_q1/3(apol) -> Mux2/1
  Mux/1 -> q_fin/1
  Mux1/1 -> dq_fin/1
  Mux2/1 -> ddq_fin/1

== system control_pos_3dof_sinMI/Inicializar posición de robot manipulador/q_init_tr ==
  q_init : Inport
  q_fin : Inport  Port=2
  t_fin : Inport  Port=3
  Demux : Demux  Outputs=3
  Demux1 : Demux  Outputs=3
  Mux : Mux  Inputs=3
  Mux1 : Mux  Inputs=3
  Mux2 : Mux  Inputs=3
  q1 : Subsystem
  q2 : Subsystem
  q3 : Subsystem
  qpol : Outport
  vpol : Outport  Port=2
  apol : Outport  Port=3
  wires:
  q_fin/1 -> Demux/1
  t_fin/1 -> [t_fin]
  [t_fin] -> q1/3(t_fin)
  [t_fin] -> q2/3(t_fin)
  [t_fin] -> q3/3(t_fin)
  Mux/1 -> qpol/1
  Demux/1 -> q1/2(q_fin)
  Demux/2 -> q2/2(q_fin)
  Demux/3 -> q3/2(q_fin)
  q1/1(qpol) -> Mux/1
  q_init/1 -> Demux1/1
  Demux1/1 -> q1/1(q_init)
  Demux1/2 -> q2/1(q_init)
  Demux1/3 -> q3/1(q_init)
  q2/1(qpol) -> Mux/2
  q3/1(qpol) -> Mux/3
  Mux1/1 -> vpol/1
  Mux2/1 -> apol/1
  q1/2(vpol) -> Mux1/1
  q2/2(vpol) -> Mux1/2
  q3/2(vpol) -> Mux1/3
  q1/3(apol) -> Mux2/1
  q2/3(apol) -> Mux2/2
  q3/3(apol) -> Mux2/3

== system control_pos_3dof_sinMI/Inicializar posición de robot manipulador/dq_init/q1 ==
  q_fin : Inport
  t_fin : Inport  Port=2
  Clock1 : Clock
  Constant : Constant  Value=pi/4
  Constant4 : Constant  Value=0
  Polinomio 7mo orden dq : MATLAB Function  TreatAsAtomicUnit=on
  Sum : Sum  Inputs=|++
  qpol : Outport
  wires:
  Clock1/1 -> Polinomio 7mo orden dq/1(t)
  Constant4/1 -> Polinomio 7mo orden dq/2(q0)
  q_fin/1 -> Polinomio 7mo orden dq/3(q1)
  t_fin/1 -> Sum/1, Polinomio 7mo orden dq/4(t0)
  Polinomio 7mo orden dq/1(qpol) -> qpol/1
  Constant/1 -> Sum/2
  Sum/1 -> Polinomio 7mo orden dq/5(t1)

== system control_pos_3dof_sinMI/Inicializar posición de robot manipulador/dq_init/q2 ==
  q_fin : Inport
  t_fin : Inport  Port=2
  Clock1 : Clock
  Constant : Constant  Value=pi/4
  Constant4 : Constant  Value=0
  Polinomio 7mo orden dq : MATLAB Function  TreatAsAtomicUnit=on
  Sum : Sum  Inputs=|++
  qpol : Outport
  wires:
  Clock1/1 -> Polinomio 7mo orden dq/1(t)
  Constant4/1 -> Polinomio 7mo orden dq/2(q0)
  q_fin/1 -> Polinomio 7mo orden dq/3(q1)
  t_fin/1 -> Sum/1, Polinomio 7mo orden dq/4(t0)
  Polinomio 7mo orden dq/1(qpol) -> qpol/1
  Constant/1 -> Sum/2
  Sum/1 -> Polinomio 7mo orden dq/5(t1)

== system control_pos_3dof_sinMI/Inicializar posición de robot manipulador/dq_init/q3 ==
  q_fin : Inport
  t_fin : Inport  Port=2
  Clock1 : Clock
  Constant : Constant  Value=pi/4
  Constant4 : Constant  Value=0
  Polinomio 7mo orden dq : MATLAB Function  TreatAsAtomicUnit=on
  Sum : Sum  Inputs=|++
  qpol : Outport
  wires:
  Clock1/1 -> Polinomio 7mo orden dq/1(t)
  Constant4/1 -> Polinomio 7mo orden dq/2(q0)
  q_fin/1 -> Polinomio 7mo orden dq/3(q1)
  t_fin/1 -> Sum/1, Polinomio 7mo orden dq/4(t0)
  Polinomio 7mo orden dq/1(qpol) -> qpol/1
  Constant/1 -> Sum/2
  Sum/1 -> Polinomio 7mo orden dq/5(t1)

== system control_pos_3dof_sinMI/Inicializar posición de robot manipulador/dq_init1/q1 ==
  q_fin : Inport
  t_fin : Inport  Port=2
  Clock1 : Clock
  Constant : Constant  Value=pi/4
  Constant4 : Constant  Value=0
  Polinomio 7mo orden dq : MATLAB Function  TreatAsAtomicUnit=on
  Sum : Sum  Inputs=|++
  qpol : Outport
  wires:
  Clock1/1 -> Polinomio 7mo orden dq/1(t)
  Constant4/1 -> Polinomio 7mo orden dq/2(q0)
  q_fin/1 -> Polinomio 7mo orden dq/3(q1)
  t_fin/1 -> Sum/1, Polinomio 7mo orden dq/4(t0)
  Polinomio 7mo orden dq/1(qpol) -> qpol/1
  Constant/1 -> Sum/2
  Sum/1 -> Polinomio 7mo orden dq/5(t1)

== system control_pos_3dof_sinMI/Inicializar posición de robot manipulador/dq_init1/q2 ==
  q_fin : Inport
  t_fin : Inport  Port=2
  Clock1 : Clock
  Constant : Constant  Value=pi/4
  Constant4 : Constant  Value=0
  Polinomio 7mo orden dq : MATLAB Function  TreatAsAtomicUnit=on
  Sum : Sum  Inputs=|++
  qpol : Outport
  wires:
  Clock1/1 -> Polinomio 7mo orden dq/1(t)
  Constant4/1 -> Polinomio 7mo orden dq/2(q0)
  q_fin/1 -> Polinomio 7mo orden dq/3(q1)
  t_fin/1 -> Sum/1, Polinomio 7mo orden dq/4(t0)
  Polinomio 7mo orden dq/1(qpol) -> qpol/1
  Constant/1 -> Sum/2
  Sum/1 -> Polinomio 7mo orden dq/5(t1)

== system control_pos_3dof_sinMI/Inicializar posición de robot manipulador/dq_init1/q3 ==
  q_fin : Inport
  t_fin : Inport  Port=2
  Clock1 : Clock
  Constant : Constant  Value=pi/4
  Constant4 : Constant  Value=0
  Polinomio 7mo orden dq : MATLAB Function  TreatAsAtomicUnit=on
  Sum : Sum  Inputs=|++
  qpol : Outport
  wires:
  Clock1/1 -> Polinomio 7mo orden dq/1(t)
  Constant4/1 -> Polinomio 7mo orden dq/2(q0)
  q_fin/1 -> Polinomio 7mo orden dq/3(q1)
  t_fin/1 -> Sum/1, Polinomio 7mo orden dq/4(t0)
  Polinomio 7mo orden dq/1(qpol) -> qpol/1
  Constant/1 -> Sum/2
  Sum/1 -> Polinomio 7mo orden dq/5(t1)

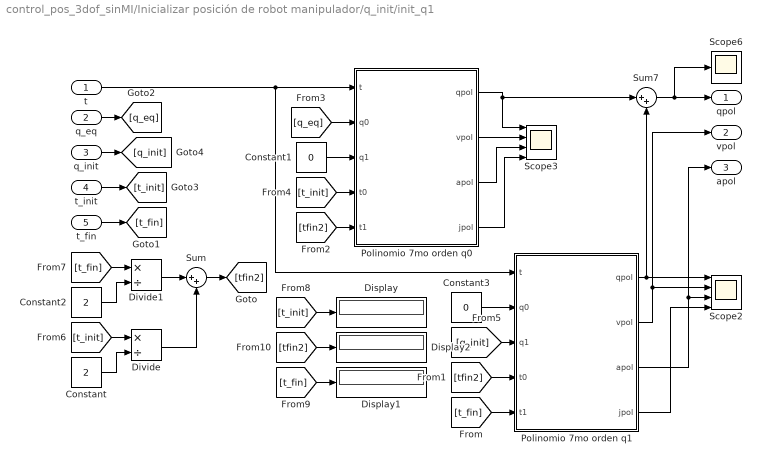
== system control_pos_3dof_sinMI/Inicializar posición de robot manipulador/q_init/init_q1 ==
  t : Inport
  q_eq : Inport  Port=2
  q_init : Inport  Port=3
  t_init : Inport  Port=4
  t_fin : Inport  Port=5
  Constant : Constant  Value=2
  Constant1 : Constant  Value=0
  Constant2 : Constant  Value=2
  Constant3 : Constant  Value=0
  Display : Display
  Display1 : Display
  Display2 : Display
  Divide : Product  Inputs=*/
  Divide1 : Product  Inputs=*/
  Polinomio 7mo orden q0 : MATLAB Function  TreatAsAtomicUnit=on
  Polinomio 7mo orden q1 : MATLAB Function  TreatAsAtomicUnit=on
  Scope2 : Scope  NumInputPorts=4
  Scope3 : Scope  NumInputPorts=4
  Scope6 : Scope
  Sum : Sum  Inputs=|++
  Sum7 : Sum  Inputs=|++
  qpol : Outport
  vpol : Outport  Port=2
  apol : Outport  Port=3
  wires:
  [tfin2] -> Polinomio 7mo orden q0/5(t1)
  t/1 -> Polinomio 7mo orden q1/1(t), Polinomio 7mo orden q0/1(t)
  t_fin/1 -> [t_fin]
  Polinomio 7mo orden q0/1(qpol) -> Sum7/1, Scope3/1
  Polinomio 7mo orden q1/1(qpol) -> Scope2/1, Sum7/2
  [tfin2] -> Polinomio 7mo orden q1/4(t0)
  [t_fin] -> Polinomio 7mo orden q1/5(t1)
  q_eq/1 -> [q_eq]
  q_init/1 -> [q_init]
  [q_eq] -> Polinomio 7mo orden q0/2(q0)
  [q_init] -> Polinomio 7mo orden q1/3(q1)
  Constant1/1 -> Polinomio 7mo orden q0/3(q1)
  Constant3/1 -> Polinomio 7mo orden q1/2(q0)
  Sum7/1 -> qpol/1, Scope6/1
  t_init/1 -> [t_init]
  [t_init] -> Polinomio 7mo orden q0/4(t0)
  Sum/1 -> [tfin2]
  [t_init] -> Display/1
  [t_fin] -> Display1/1
  [tfin2] -> Display2/1
  Divide/1 -> Sum/2
  Constant/1 -> Divide/2
  Divide1/1 -> Sum/1
  Constant2/1 -> Divide1/2
  [t_fin] -> Divide1/1
  [t_init] -> Divide/1
  Polinomio 7mo orden q1/2(vpol) -> vpol/1, Scope2/2
  Polinomio 7mo orden q1/3(apol) -> apol/1, Scope2/3
  Polinomio 7mo orden q1/4(jpol) -> Scope2/4
  Polinomio 7mo orden q0/2(vpol) -> Scope3/2
  Polinomio 7mo orden q0/3(apol) -> Scope3/3
  Polinomio 7mo orden q0/4(jpol) -> Scope3/4

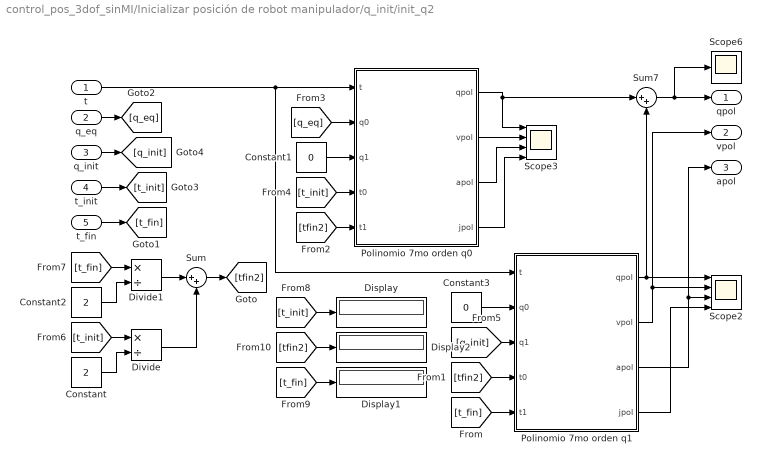
== system control_pos_3dof_sinMI/Inicializar posición de robot manipulador/q_init/init_q2 ==
  t : Inport
  q_eq : Inport  Port=2
  q_init : Inport  Port=3
  t_init : Inport  Port=4
  t_fin : Inport  Port=5
  Constant : Constant  Value=2
  Constant1 : Constant  Value=0
  Constant2 : Constant  Value=2
  Constant3 : Constant  Value=0
  Display : Display
  Display1 : Display
  Display2 : Display
  Divide : Product  Inputs=*/
  Divide1 : Product  Inputs=*/
  Polinomio 7mo orden q0 : MATLAB Function  TreatAsAtomicUnit=on
  Polinomio 7mo orden q1 : MATLAB Function  TreatAsAtomicUnit=on
  Scope2 : Scope  NumInputPorts=4
  Scope3 : Scope  NumInputPorts=4
  Scope6 : Scope
  Sum : Sum  Inputs=|++
  Sum7 : Sum  Inputs=|++
  qpol : Outport
  vpol : Outport  Port=2
  apol : Outport  Port=3
  wires:
  [tfin2] -> Polinomio 7mo orden q0/5(t1)
  t/1 -> Polinomio 7mo orden q1/1(t), Polinomio 7mo orden q0/1(t)
  t_fin/1 -> [t_fin]
  Polinomio 7mo orden q0/1(qpol) -> Sum7/1, Scope3/1
  Polinomio 7mo orden q1/1(qpol) -> Scope2/1, Sum7/2
  [tfin2] -> Polinomio 7mo orden q1/4(t0)
  [t_fin] -> Polinomio 7mo orden q1/5(t1)
  q_eq/1 -> [q_eq]
  q_init/1 -> [q_init]
  [q_eq] -> Polinomio 7mo orden q0/2(q0)
  [q_init] -> Polinomio 7mo orden q1/3(q1)
  Constant1/1 -> Polinomio 7mo orden q0/3(q1)
  Constant3/1 -> Polinomio 7mo orden q1/2(q0)
  Sum7/1 -> qpol/1, Scope6/1
  t_init/1 -> [t_init]
  [t_init] -> Polinomio 7mo orden q0/4(t0)
  Sum/1 -> [tfin2]
  [t_init] -> Display/1
  [t_fin] -> Display1/1
  [tfin2] -> Display2/1
  Divide/1 -> Sum/2
  Constant/1 -> Divide/2
  Divide1/1 -> Sum/1
  Constant2/1 -> Divide1/2
  [t_fin] -> Divide1/1
  [t_init] -> Divide/1
  Polinomio 7mo orden q1/2(vpol) -> vpol/1, Scope2/2
  Polinomio 7mo orden q1/3(apol) -> apol/1, Scope2/3
  Polinomio 7mo orden q1/4(jpol) -> Scope2/4
  Polinomio 7mo orden q0/2(vpol) -> Scope3/2
  Polinomio 7mo orden q0/3(apol) -> Scope3/3
  Polinomio 7mo orden q0/4(jpol) -> Scope3/4

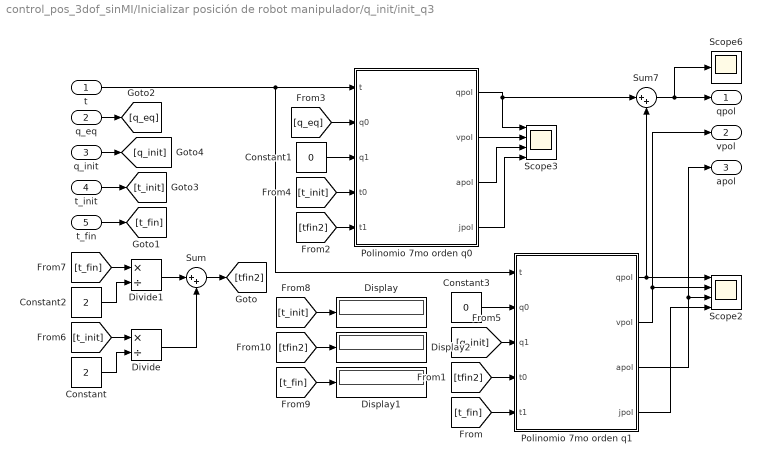
== system control_pos_3dof_sinMI/Inicializar posición de robot manipulador/q_init/init_q3 ==
  t : Inport
  q_eq : Inport  Port=2
  q_init : Inport  Port=3
  t_init : Inport  Port=4
  t_fin : Inport  Port=5
  Constant : Constant  Value=2
  Constant1 : Constant  Value=0
  Constant2 : Constant  Value=2
  Constant3 : Constant  Value=0
  Display : Display
  Display1 : Display
  Display2 : Display
  Divide : Product  Inputs=*/
  Divide1 : Product  Inputs=*/
  Polinomio 7mo orden q0 : MATLAB Function  TreatAsAtomicUnit=on
  Polinomio 7mo orden q1 : MATLAB Function  TreatAsAtomicUnit=on
  Scope2 : Scope  NumInputPorts=4
  Scope3 : Scope  NumInputPorts=4
  Scope6 : Scope
  Sum : Sum  Inputs=|++
  Sum7 : Sum  Inputs=|++
  qpol : Outport
  vpol : Outport  Port=2
  apol : Outport  Port=3
  wires:
  [tfin2] -> Polinomio 7mo orden q0/5(t1)
  t/1 -> Polinomio 7mo orden q1/1(t), Polinomio 7mo orden q0/1(t)
  t_fin/1 -> [t_fin]
  Polinomio 7mo orden q0/1(qpol) -> Sum7/1, Scope3/1
  Polinomio 7mo orden q1/1(qpol) -> Scope2/1, Sum7/2
  [tfin2] -> Polinomio 7mo orden q1/4(t0)
  [t_fin] -> Polinomio 7mo orden q1/5(t1)
  q_eq/1 -> [q_eq]
  q_init/1 -> [q_init]
  [q_eq] -> Polinomio 7mo orden q0/2(q0)
  [q_init] -> Polinomio 7mo orden q1/3(q1)
  Constant1/1 -> Polinomio 7mo orden q0/3(q1)
  Constant3/1 -> Polinomio 7mo orden q1/2(q0)
  Sum7/1 -> qpol/1, Scope6/1
  t_init/1 -> [t_init]
  [t_init] -> Polinomio 7mo orden q0/4(t0)
  Sum/1 -> [tfin2]
  [t_init] -> Display/1
  [t_fin] -> Display1/1
  [tfin2] -> Display2/1
  Divide/1 -> Sum/2
  Constant/1 -> Divide/2
  Divide1/1 -> Sum/1
  Constant2/1 -> Divide1/2
  [t_fin] -> Divide1/1
  [t_init] -> Divide/1
  Polinomio 7mo orden q1/2(vpol) -> vpol/1, Scope2/2
  Polinomio 7mo orden q1/3(apol) -> apol/1, Scope2/3
  Polinomio 7mo orden q1/4(jpol) -> Scope2/4
  Polinomio 7mo orden q0/2(vpol) -> Scope3/2
  Polinomio 7mo orden q0/3(apol) -> Scope3/3
  Polinomio 7mo orden q0/4(jpol) -> Scope3/4

== system control_pos_3dof_sinMI/Inicializar posición de robot manipulador/q_init_tr/q1 ==
  q_init : Inport
  q_fin : Inport  Port=2
  t_fin : Inport  Port=3
  Clock1 : Clock
  Constant : Constant  Value=pi/4
  Polinomio 7mo orden dq : MATLAB Function  TreatAsAtomicUnit=on
  Sum : Sum  Inputs=|++
  qpol : Outport
  vpol : Outport  Port=2
  apol : Outport  Port=3
  wires:
  Clock1/1 -> Polinomio 7mo orden dq/1(t)
  q_fin/1 -> Polinomio 7mo orden dq/3(q1)
  t_fin/1 -> Sum/1, Polinomio 7mo orden dq/4(t0)
  Polinomio 7mo orden dq/1(qpol) -> qpol/1
  Constant/1 -> Sum/2
  Sum/1 -> Polinomio 7mo orden dq/5(t1)
  q_init/1 -> Polinomio 7mo orden dq/2(q0)
  Polinomio 7mo orden dq/2(vpol) -> vpol/1
  Polinomio 7mo orden dq/3(apol) -> apol/1

== system control_pos_3dof_sinMI/Inicializar posición de robot manipulador/q_init_tr/q2 ==
  q_init : Inport
  q_fin : Inport  Port=2
  t_fin : Inport  Port=3
  Clock1 : Clock
  Constant : Constant  Value=pi/4
  Polinomio 7mo orden dq : MATLAB Function  TreatAsAtomicUnit=on
  Sum : Sum  Inputs=|++
  qpol : Outport
  vpol : Outport  Port=2
  apol : Outport  Port=3
  wires:
  Clock1/1 -> Polinomio 7mo orden dq/1(t)
  q_fin/1 -> Polinomio 7mo orden dq/3(q1)
  t_fin/1 -> Sum/1, Polinomio 7mo orden dq/4(t0)
  Polinomio 7mo orden dq/1(qpol) -> qpol/1
  Constant/1 -> Sum/2
  Sum/1 -> Polinomio 7mo orden dq/5(t1)
  q_init/1 -> Polinomio 7mo orden dq/2(q0)
  Polinomio 7mo orden dq/2(vpol) -> vpol/1
  Polinomio 7mo orden dq/3(apol) -> apol/1

== system control_pos_3dof_sinMI/Inicializar posición de robot manipulador/q_init_tr/q3 ==
  q_init : Inport
  q_fin : Inport  Port=2
  t_fin : Inport  Port=3
  Clock1 : Clock
  Constant : Constant  Value=pi/4
  Polinomio 7mo orden dq : MATLAB Function  TreatAsAtomicUnit=on
  Sum : Sum  Inputs=|++
  qpol : Outport
  vpol : Outport  Port=2
  apol : Outport  Port=3
  wires:
  Clock1/1 -> Polinomio 7mo orden dq/1(t)
  q_fin/1 -> Polinomio 7mo orden dq/3(q1)
  t_fin/1 -> Sum/1, Polinomio 7mo orden dq/4(t0)
  Polinomio 7mo orden dq/1(qpol) -> qpol/1
  Constant/1 -> Sum/2
  Sum/1 -> Polinomio 7mo orden dq/5(t1)
  q_init/1 -> Polinomio 7mo orden dq/2(q0)
  Polinomio 7mo orden dq/2(vpol) -> vpol/1
  Polinomio 7mo orden dq/3(apol) -> apol/1

== matlab function control_pos_3dof_sinMI/xyz to q (referencia)/dr to dq ==
  data: JPinv input size=[3,3]; dq output size=[3,1]; dr input size=[3,1]
function dq = fcn(JPinv,dr)

% Velocidades articulares
dq = JPinv*dr;

== matlab function control_pos_3dof_sinMI/xyz to q (referencia)/Jacobiano inverso ==
  data: robot_params input; q input size=[3,1]; JPinv output size=[3,3]
function JPinv = JPinv(robot_params,q)

l2 = robot_params.l(2);
l3 = robot_params.l(3);

q1 = q(1);
q2 = q(2);
q3 = q(3);

% Cinematica diferencial %%%%%%%%%%%%%%%%%%%%%%%%%%%%%%%%%%%%%%%%%%%%%%%%%%

JPinv = zeros(3,3);
JPinv(1,1) = -sin(q1)/(l2*cos(q2) + l3*cos(q2 + q3));
JPinv(1,2) = cos(q1)/(l2*cos(q2) + l3*cos(q2 + q3));

JPinv(2,1) = cos(q1)*cos(q2 + q3)/(l2*sin(q3));
JPinv(2,2) = sin(q1)*cos(q2 + q3)/(l2*sin(q3));
JPinv(2,3) = sin(q2 + q3)/(l2*sin(q3));

JPinv(3,1) = -(cos(q1)*(l2*cos(q2) + l3*cos(q2 + q3)))/(l2*l3*sin(q3));
JPinv(3,2) = -(sin(q1)*(l2*cos(q2) + l3*cos(q2 + q3)))/(l2*l3*sin(q3));
JPinv(3,3) = -(l2*sin(q2) + l3*sin(q2 + q3))/(l2*l3*sin(q3));

== matlab function control_pos_3dof_sinMI/xyz to q (referencia)/derivada Jacobiano ==
  data: robot_params input; q input size=[3,1]; dJP output size=[3,3]; dq input size=[3,1]
function dJP = dJP(robot_params,q,dq)

l2 = robot_params.l(2);
l3 = robot_params.l(3);

dq1 = dq(1);
dq2 = dq(2);
dq3 = dq(3);


q1 = q(1);
q2 = q(2);
q3 = q(3);

dJP = zeros(3,3);

dJP(1,1) = - cos(q1)*(l2*cos(q2) + l3*cos(q2 + q3))*dq1 + sin(q1)*(l2*sin(q2) + l3*sin(q2 + q3))*dq2 + l3*sin(q1)*sin(q2 + q3)*dq3;
dJP(1,2) =   sin(q1)*(l2*sin(q2) + l3*sin(q2 + q3))*dq1 - cos(q1)*(l2*cos(q2) + l3*cos(q2 + q3))*dq2 - l3*cos(q1)*cos(q2 + q3)*dq3;
dJP(1,3) =   l3*sin(q1)*sin(q2 + q3)*dq1 - l3*cos(q1)*cos(q2 + q3)*dq2 - l3*cos(q1)*cos(q2 + q3)*dq3;

dJP(2,1) = - sin(q1)*(l2*cos(q2) + l3*cos(q2 + q3))*dq1 - cos(q1)*(l2*sin(q2) + l3*sin(q2 + q3))*dq2 - l3*cos(q1)*sin(q2 + q3)*dq3;
dJP(2,2) = - cos(q1)*(l2*sin(q2) + l3*sin(q2 + q3))*dq1 - sin(q1)*(l2*cos(q2) + l3*cos(q2 + q3))*dq2 - l3*sin(q1)*cos(q2 + q3)*dq3;
dJP(2,3) = - l3*cos(q1)*sin(q2 + q3)*dq1 - l3*sin(q1)*cos(q2 + q3)*dq2 - l3*sin(q1)*cos(q2 + q3)*dq3;

dJP(3,1) = 0;
dJP(3,2) = - (l2*sin(q2) + l3*sin(q2 + q3))*dq2 - l3*sin(q2 + q3)*dq3;
dJP(3,3) = - l3*sin(q2 + q3)*(dq2 + dq3);

== matlab function control_pos_3dof_sinMI/xyz to q (referencia)/ddr to ddq ==
  data: JPinv input size=[3,3]; ddq output size=[3,1]; dJP input size=[3,3]; dq input size=[3,1]; ddr input size=[3,1]
function ddq = fcn(JPinv,dJP,dq,ddr)

% Aceleraciones articulares
ddq = JPinv*(ddr - dJP*dq);

== matlab function control_pos_3dof_sinMI/Dinámica inversa (referencia)/Modelo dinámico ==
  data: robot_params input; robot_din output Bus: robot_din_bus size=1; q input size=[3,1]; dq input size=[3,1]
function robot_din = fcn(robot_params,q,dq)

%d1 = robot_params.d(1);
l2 = robot_params.l(2);
lc2 = robot_params.lc(2);
%l3 = robot_params.l(3);
lc3 = robot_params.lc(3);

%m1 = robot_params.m(1);
m2 = robot_params.m(2);
m3 = robot_params.m(3);

Iz1 = robot_params.I(1,3);
Iy2 = robot_params.I(2,2);
Iz2 = robot_params.I(2,3);
Iy3 = robot_params.I(3,2);
Iz3 = robot_params.I(3,3);

g = 9.81;

q1 = q(1);
q2 = q(2);
q3 = q(3);

dq1 = dq(1);
dq2 = dq(2);
dq3 = dq(3);

D = zeros(3,3);

D(1,1) = Iz1 + Iz2 + Iz3 + (m2/2)*lc2^2*(1+cos(2*q2)) ...
       + (m3/2)*(l2^2*(1+cos(2*q2)) + 2*l2*lc3*(cos(2*q2+q3)+cos(q3)) ...
       + lc3^2*(1+cos(2*q2+2*q3)));

D(2,2) = Iy2 + Iy3 + m2*lc2^2 + m3*(l2^2 + 2*l2*lc3*cos(q3) + lc3^2);
D(2,3) = Iy3 + m3*(l2*lc3*cos(q3) + lc3^2);

D(3,2) = Iy3 + m3*(l2*lc3*cos(q3) + lc3^2);
D(3,3) = Iy3 + m3*lc3^2;

C = zeros(3,3);

C(1,2) = - ((m2*lc2^2*sin(2*q2)) ...
         + m3*(l2^2*sin(2*q2) + 2*l2*lc3*sin(2*q2+q3) ...
         + lc3^2*sin(2*q2+2*q3)))*dq1;
C(1,3) = - m3*(l2*lc3*(sin(2*q2+q3)+sin(q3)) ...
         + lc3^2*(sin(2*q2+2*q3)))*dq1;

C(2,1) =   ((m2/2)*(lc2^2*sin(2*q2)) ...
         + (m3/2)*(l2^2*sin(2*q2) + 2*l2*lc3*sin(2*q2+q3) ...
         + lc3^2*sin(2*q2+2*q3)))*dq1;
C(2,2) = - 2*m3*l2*lc3*sin(q3)*dq3;
C(2,3) = - m3*l2*lc3*sin(q3)*dq3;

C(3,1) =   (m3/2)*(l2*lc3*(sin(2*q2+q3) + sin(q3)) ...
         + lc3^2*sin(2*q2+2*q3))*dq1;
C(3,2) =   m3*l2*lc3*sin(q3)*dq2;

G = zeros(3,1);

G(2,1) = m2*lc2*cos(q2) + m3*(l2*cos(q2) + lc3*cos(q2+q3));
G(3,1) = m3*lc3*cos(q2+q3);


robot_din = struct('D',D,'C',C,'G',G,'g',9.81);

%busInfo = Simulink.Bus.createObject(robot_dyn);

== matlab function control_pos_3dof_sinMI/Dinámica inversa (referencia)/Dinámica inversa ==
  data: robot_din input; dq input size=[3,1]; tau_s output size=[3,1]; ddq input size=[3,1]
function tau_s = fcn(robot_din,dq,ddq)

D = robot_din.D;
C = robot_din.C;
G = robot_din.G;
g = robot_din.g;

tau_s = D*ddq + C*dq + G*g;

== matlab function control_pos_3dof_sinMI/q to xyz (referencia)/derivada Jacobiano ==
  data: robot_params input; q input size=[3,1]; dJP output size=[3,3]; dq input size=[3,1]
function dJP = dJP(robot_params,q,dq)

l2 = robot_params.l(2);
l3 = robot_params.l(3);

dq1 = dq(1);
dq2 = dq(2);
dq3 = dq(3);


q1 = q(1);
q2 = q(2);
q3 = q(3);

dJP = zeros(3,3);

dJP(1,1) = - cos(q1)*(l2*cos(q2) + l3*cos(q2 + q3))*dq1 + sin(q1)*(l2*sin(q2) + l3*sin(q2 + q3))*dq2 + l3*sin(q1)*sin(q2 + q3)*dq3;
dJP(1,2) =   sin(q1)*(l2*sin(q2) + l3*sin(q2 + q3))*dq1 - cos(q1)*(l2*cos(q2) + l3*cos(q2 + q3))*dq2 - l3*cos(q1)*cos(q2 + q3)*dq3;
dJP(1,3) =   l3*sin(q1)*sin(q2 + q3)*dq1 - l3*cos(q1)*cos(q2 + q3)*dq2 - l3*cos(q1)*cos(q2 + q3)*dq3;

dJP(2,1) = - sin(q1)*(l2*cos(q2) + l3*cos(q2 + q3))*dq1 - cos(q1)*(l2*sin(q2) + l3*sin(q2 + q3))*dq2 - l3*cos(q1)*sin(q2 + q3)*dq3;
dJP(2,2) = - cos(q1)*(l2*sin(q2) + l3*sin(q2 + q3))*dq1 - sin(q1)*(l2*cos(q2) + l3*cos(q2 + q3))*dq2 - l3*sin(q1)*cos(q2 + q3)*dq3;
dJP(2,3) = - l3*cos(q1)*sin(q2 + q3)*dq1 - l3*sin(q1)*cos(q2 + q3)*dq2 - l3*sin(q1)*cos(q2 + q3)*dq3;

dJP(3,1) = 0;
dJP(3,2) = - (l2*sin(q2) + l3*sin(q2 + q3))*dq2 - l3*sin(q2 + q3)*dq3;
dJP(3,3) = - l3*sin(q2 + q3)*(dq2 + dq3);

== matlab function control_pos_3dof_sinMI/q to xyz (referencia)/Cinemática directa ==
  data: robot_params input; p output size=[3,3]; q input size=[3,1]
function p  = fcn(robot_params,q)

d1 = robot_params.d(1);
l2 = robot_params.l(2);
l3 = robot_params.l(3);

q1 = q(1);
q2 = q(2);
q3 = q(3);

p1 = [0;0;d1];

p2 = [l2*cos(q1)*cos(q2);
      l2*sin(q1)*cos(q2);
      d1+l2*sin(q2)];

p3 = [cos(q1)*(l2*cos(q2)+l3*cos(q2+q3));
      sin(q1)*(l2*cos(q2)+l3*cos(q2+q3));
      d1+l2*sin(q2)+l3*sin(q2+q3)];

p = [p1,p2,p3];

== matlab function control_pos_3dof_sinMI/q to xyz (referencia)/Jacobiano ==
  data: robot_params input; JP output size=[3,3]; q input size=[3,1]
function JP = fcn(robot_params,q)

l2 = robot_params.l(2);
l3 = robot_params.l(3);

q1 = q(1);
q2 = q(2);
q3 = q(3);

JP = zeros(3,3);

JP(1,1) = -sin(q1)*(l2*cos(q2) + l3*cos(q2 + q3));
JP(1,2) = -cos(q1)*(l2*sin(q2) + l3*sin(q2 + q3));
JP(1,3) = -l3*cos(q1)*sin(q2 + q3);

JP(2,1) =  cos(q1)*(l2*cos(q2) + l3*cos(q2 + q3));
JP(2,2) = -sin(q1)*(l2*sin(q2) + l3*sin(q2 + q3));
JP(2,3) = -l3*sin(q1)*sin(q2 + q3);

JP(3,2) = l2*cos(q2) + l3*cos(q2 + q3);
JP(3,3) = l3*cos(q2 + q3);
